simulink model "harness"  (R2024b)
settings: Solver=VariableStepAuto  StartTime=0.0  StopTime=30  RelTol=1e-3
undefined symbols (not defined in the file): matlabshared
libraries: drivingscenarioandsensors x3, autolibshared x1
settings Model: DataDictionary=data.sldd  EnableAccessToBaseWorkspace=off  Creator=maciej  LastModifiedBy=maciej

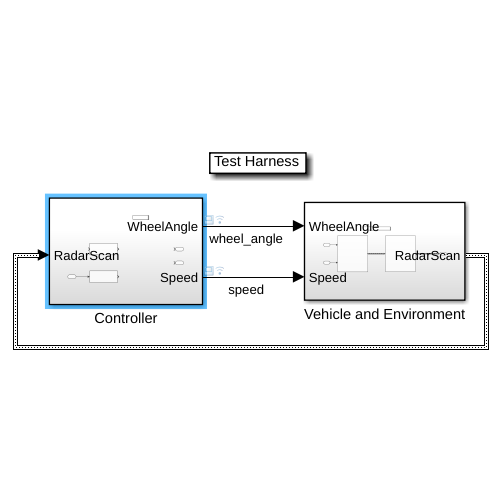
[thumbnail: Simulink's stored preview of the top-level diagram]
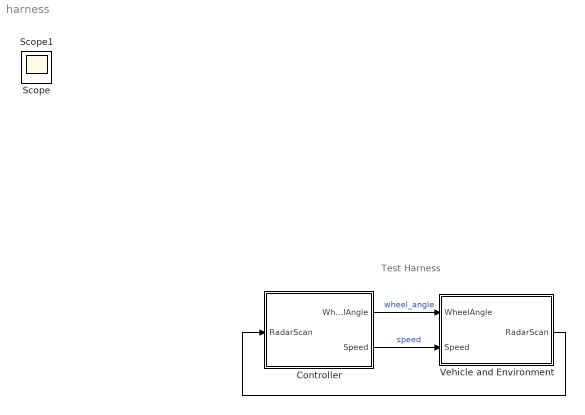
== system harness ==
  note: Test Harness
  Controller : Subsystem
  Vehicle and Environment : Subsystem
  Scope : Scope
  Scope1 : Scope
  wires:
  Vehicle and Environment/1(RadarScan) -> Controller/1(RadarScan)
  Controller/1(WheelAngle) -> Vehicle and Environment/1(WheelAngle)  "wheel_angle"
  Controller/2(Speed) -> Vehicle and Environment/2(Speed)  "speed"

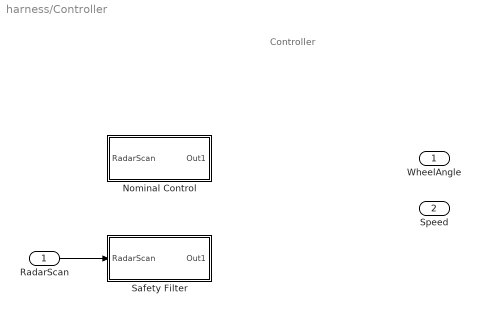
== system harness/Controller ==
  note: Controller
  RadarScan : Inport
  Nominal Control : Subsystem
  Safety Filter : Subsystem
  WheelAngle : Outport
  Speed : Outport  Port=2
  wires:
  RadarScan/1 -> Safety Filter/1(RadarScan)

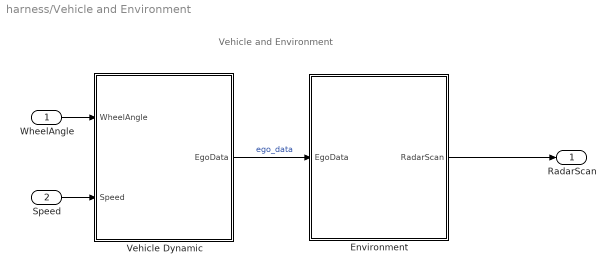
== system harness/Vehicle and Environment ==
  note: Vehicle and Environment
  WheelAngle : Inport
  Speed : Inport  Port=2
  Environment : Subsystem
  Vehicle Dynamic : Subsystem
  RadarScan : Outport
  wires:
  WheelAngle/1 -> Vehicle Dynamic/1(WheelAngle)
  Speed/1 -> Vehicle Dynamic/2(Speed)
  Vehicle Dynamic/1(EgoData) -> Environment/1(EgoData)  "ego_data"
  Environment/1(RadarScan) -> RadarScan/1

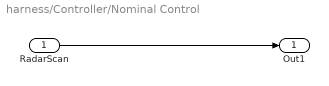
== system harness/Controller/Nominal Control ==
  RadarScan : Inport
  Out1 : Outport
  wires:
  RadarScan/1 -> Out1/1

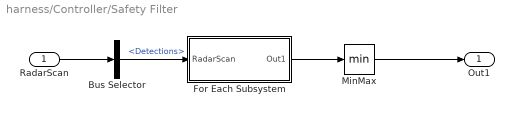
== system harness/Controller/Safety Filter ==
  RadarScan : Inport
  Bus Selector : BusSelector  OutputSignals=Detections
  For Each Subsystem : Subsystem  TreatAsAtomicUnit=on
  MinMax : MinMax
  Out1 : Outport
  wires:
  RadarScan/1 -> Bus Selector/1
  Bus Selector/1 -> For Each Subsystem/1(RadarScan)  "<Detections>"
  For Each Subsystem/1(Out1) -> MinMax/1
  MinMax/1 -> Out1/1

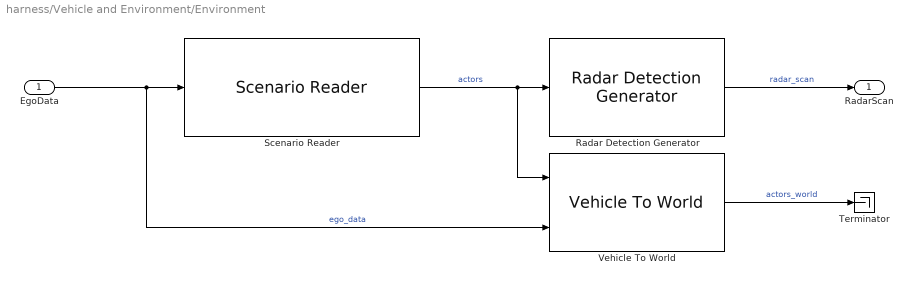
== system harness/Vehicle and Environment/Environment ==
  EgoData : Inport
  Radar Detection Generator : drivingscenarioandsensors/Radar Detection Generator  SensorIndex=1  UpdateInterval=0.1  SensorLocation=[ 3.4, 0 ]  Height=0.2  Yaw=0  Pitch=0  Roll=0  BusNameSource=Auto  BusName=BusRadarDetectionGenerator  MaxNumDetectionsSource=Property  MaxNumDetections=50  DetectionCoordinates=Ego Cartesian  SimulateUsing=Interpreted execution  AzimuthResolution=4  ElevationResolution=10  RangeResolution=2.5  RangeRateResolution=0.5  AzimuthBiasFraction=0.1  ElevationBiasFraction=0.1  RangeBiasFraction=0.05  RangeRateBiasFraction=0.05  FieldOfView=[ 20, 5 ]  MaxRange=150  RangeRateLimits=[ -100, 100 ]  DetectionProbability=0.9  FalseAlarmRate=1e-6  ReferenceRange=100  ReferenceRCS=0  HasElevation=off  HasRangeRate=on  HasNoise=on  HasFalseAlarms=on  HasOcclusion=on  InitialSeedSource=Repeatable  InitialSeed=0  UsedSeed=matlabshared.tracking.internal.SimulinkUtilities.seedManager(gcb)  ActorProfilesSource=Parameters  ActorProfilesParameters=driving.internal.ActorProfilesRadarParameters  ActorProfilesExpression=struct( 'ClassID', 0, 'Length', 4.7, 'Width', 1.8, 'Height', 1.4, 'OriginOffset', [ -1.35, 0, 0 ], 'RCSPattern', [ 10, 10; 10, 10 ], 'RCSAzimuthAngles', [ -180, 180 ], 'RCSElevationAngles', [ -90, 90 ] )
  Scenario Reader : drivingscenarioandsensors/Scenario Reader  ScenarioSource=From file  ScenarioFileName=/home/maciej/repos/cbf_parking/scenarios/scenario_1.mat  ScenarioVariableName=scenario  OutputCoordinateSystem=Vehicle coordinates  EgoVehicleSource=Input port  EgoVehicleActorID=1  OrientVehiclesOnRoad=off  OutputEgoVehiclePose=off  OutputEgoVehicleState=off  SampleTime=0.1  LaneBoundaryOutput=None  LaneBoundaryDistance=0:0.5:9.5  LaneBoundaryLocation=Center of lane markings  BusNameSource=Auto  BusName=BusActors  BusNumActorsSource=Scenario  BusNumActors=100  BusName2Source=Auto  BusName2=BusLaneBoundaries  BusNumLaneBoundariesSource=Scenario  BusNumLaneBoundaries=10  BusName3Source=Auto  BusName3=BusEgoActor  BusName4Source=Auto  BusName4=BusEgoState  ShowCoordinateLabels=on  SimulateUsing=Interpreted execution
  Terminator : Terminator
  Vehicle To World : drivingscenarioandsensors/Vehicle To World  BusNameSource=Auto  BusName=BusVehicleToWorldActors  SimulateUsing=Interpreted execution
  RadarScan : Outport
  wires:
  EgoData/1 -> Vehicle To World/2, Scenario Reader/1  "ego_data"
  Scenario Reader/1 -> Vehicle To World/1, Radar Detection Generator/1  "actors"
  Radar Detection Generator/1 -> RadarScan/1  "radar_scan"
  Vehicle To World/1 -> Terminator/1  "actors_world"

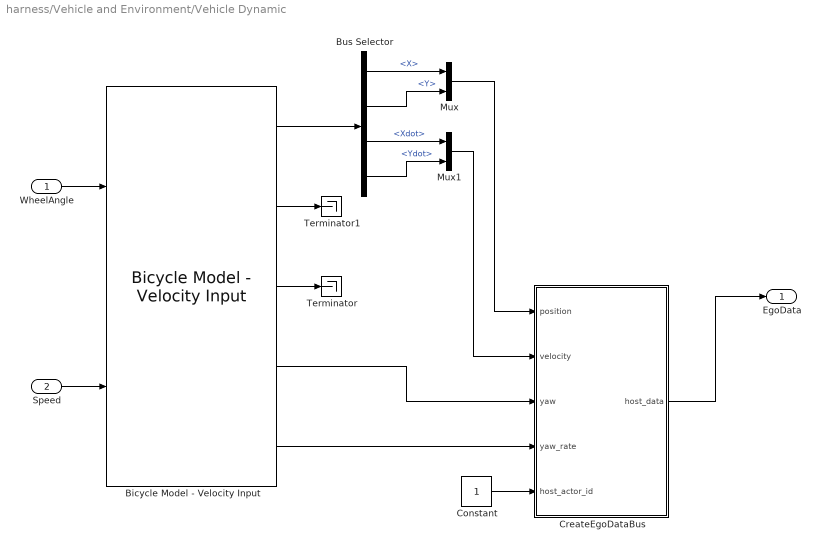
== system harness/Vehicle and Environment/Vehicle Dynamic ==
  WheelAngle : Inport
  Speed : Inport  Port=2
  Bicycle Model - Velocity Input : autolibshared/Bicycle Model - Velocity Input  trackMode=Single (bicycle)  inputMode=External longitudinal velocity  frontSteerMode=on  rearSteerMode=off  windMode=off  muMode=off  extFMode=off  extMMode=off  aMode=3  NF=2  NR=2  m=2000  a=1.4  b=1.6  h=0.35  X_o=0  xdot_o=0  CalphaMode=off  sigmaMode=on  w=[1.4,1.4]  Cy_f=12e3  Cy_r=11e3  sigma_f=.1  sigma_r=.1  alpha_f_brk=[-.1 .1]  Cy_f_data=[-9e3 9e3]  alpha_r_brk=[-.1 .1]  Cy_r_data=[-9e3 9e3]  Y_o=0  ydot_o=0  Izz=4000  psi_o=0  r_o=0  Af=2  Cd=.3  Cl=.1  Cpm=.1  beta_w=[0 0.01:0.01:0.3]  Cs=[0 0.01:0.01:0.3]  Cym=[0 1e-6:0.01:0.3]  Pabs=101325  Tair=273  g=9.81  mu=1  xdot_tol=.01  Fznom=5000  Fxtire_sat=1e6  Fytire_sat=1e6  longOff=0  latOff=0  vertOff=0
      settings: LibrarySourceBlock=drivingscenarioandsensors/Bicycle Model - Velocity Input
  Bus Selector : BusSelector  OutputSignals=InertFrm.RearAxl.Disp.X,InertFrm.RearAxl.Disp.Y,InertFrm.RearAxl.Vel.Xdot,InertFrm.RearAxl.Vel.Ydot
  Constant : Constant
  CreateEgoDataBus : MATLAB Function  TreatAsAtomicUnit=on
  Mux : Mux  Inputs=2
  Mux1 : Mux  Inputs=2
  Terminator : Terminator
  Terminator1 : Terminator
  EgoData : Outport
  wires:
  WheelAngle/1 -> Bicycle Model - Velocity Input/1
  Speed/1 -> Bicycle Model - Velocity Input/2
  Constant/1 -> CreateEgoDataBus/5(host_actor_id)
  Bicycle Model - Velocity Input/5 -> CreateEgoDataBus/4(yaw_rate)
  Bicycle Model - Velocity Input/4 -> CreateEgoDataBus/3(yaw)
  Bicycle Model - Velocity Input/3 -> Terminator/1
  Bicycle Model - Velocity Input/2 -> Terminator1/1
  Bicycle Model - Velocity Input/1 -> Bus Selector/1
  Bus Selector/1 -> Mux/1  "<X>"
  Bus Selector/2 -> Mux/2  "<Y>"
  Bus Selector/3 -> Mux1/1  "<Xdot>"
  Bus Selector/4 -> Mux1/2  "<Ydot>"
  Mux/1 -> CreateEgoDataBus/1(position)
  Mux1/1 -> CreateEgoDataBus/2(velocity)
  CreateEgoDataBus/1(host_data) -> EgoData/1

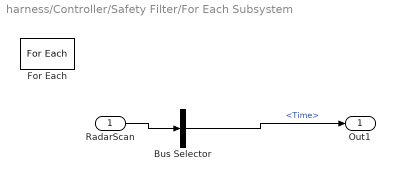
== system harness/Controller/Safety Filter/For Each Subsystem ==
  RadarScan : Inport  Partition=on  PartitionDimension=1  PartitionWidth=1  PartitionOffset=0
  Bus Selector : BusSelector  OutputSignals=Time
  For Each : ForEach  DisableCoverage=on
  Out1 : Outport  ConcatenationDimension=1
  wires:
  RadarScan/1 -> Bus Selector/1
  Bus Selector/1 -> Out1/1  "<Time>"

== matlab function harness/Vehicle and Environment/Vehicle Dynamic/CreateEgoDataBus ==
  data: position input; host_data output Bus: EgoData; velocity input; yaw input; yaw_rate input; host_actor_id input
function host_data = CreateEgoDataBus(position, velocity, yaw, yaw_rate, host_actor_id)
% Pack ego information into a single ego actor bus
%
% Imoprtant note:
% Output is a bus of type EgoData. This is the same bus used by the
% Scenario Reader to output an individual actor.

    host_data = struct(...
        'ActorID', host_actor_id,...
        'Position', [position(1) position(2) 0], ...
        'Velocity', [velocity(1) velocity(2) 0], ...
        'Roll', 0, ...
        'Pitch', 0, ...
        'Yaw', yaw, ...
        'AngularVelocity', [0 0 yaw_rate]);
end
